simulink model "heldreset"  (R2022b)
settings: Solver=FixedStepDiscrete  StartTime=0.0  StopTime=10.0  FixedStep=0.1  RelTol=1e-3
settings Model: Creator=ahmed  LastModifiedBy=ahmed

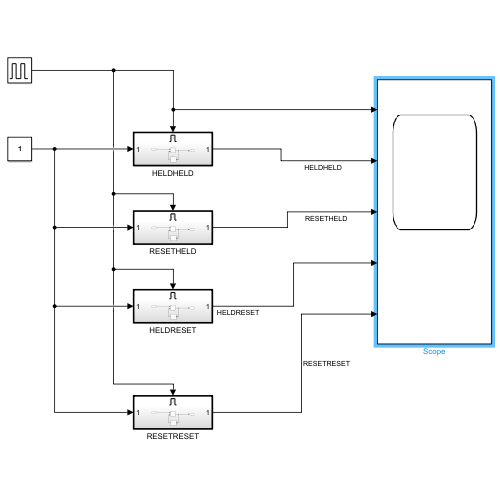
[thumbnail: Simulink's stored preview of the top-level diagram]
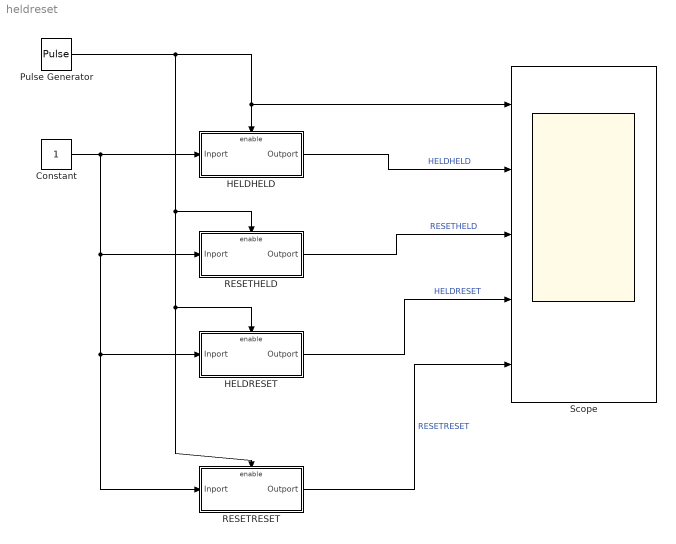
== system heldreset ==
  Constant : Constant
  HELDHELD : Subsystem  TreatAsAtomicUnit=on
  HELDRESET : Subsystem  TreatAsAtomicUnit=on
  Pulse Generator : DiscretePulseGenerator  PulseType=Time based  Period=1  PulseWidth=50
  RESETHELD : Subsystem  TreatAsAtomicUnit=on
  RESETRESET : Subsystem  TreatAsAtomicUnit=on
  Scope : Scope  NumInputPorts=5
  wires:
  Constant/1 -> HELDHELD/1(Inport), HELDRESET/1(Inport), RESETRESET/1(Inport), RESETHELD/1(Inport)
  Pulse Generator/1 -> RESETHELD/Enable, HELDRESET/Enable, RESETRESET/Enable, HELDHELD/Enable, Scope/1
  HELDHELD/1(Outport) -> Scope/2  "HELDHELD"
  RESETHELD/1(Outport) -> Scope/3  "RESETHELD"
  RESETRESET/1(Outport) -> Scope/5  "RESETRESET"
  HELDRESET/1(Outport) -> Scope/4  "HELDRESET"

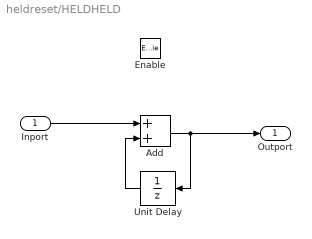
== system heldreset/HELDHELD ==
  Inport : Inport
  Enable : EnablePort
  Add : Sum
  Unit Delay : UnitDelay  SampleTime=-1  HasFrameUpgradeWarning=on
  Outport : Outport
  wires:
  Unit Delay/1 -> Add/2
  Add/1 -> Outport/1, Unit Delay/1
  Inport/1 -> Add/1

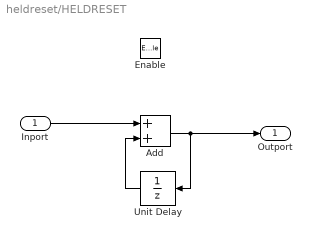
== system heldreset/HELDRESET ==
  Inport : Inport
  Enable : EnablePort
  Add : Sum
  Unit Delay : UnitDelay  SampleTime=-1  HasFrameUpgradeWarning=on
  Outport : Outport  OutputWhenDisabled=reset  InitialOutput=0
  wires:
  Inport/1 -> Add/1
  Add/1 -> Unit Delay/1, Outport/1
  Unit Delay/1 -> Add/2

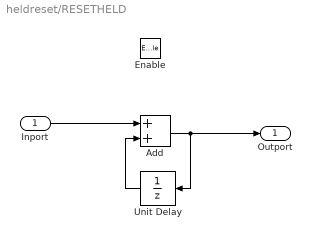
== system heldreset/RESETHELD ==
  Inport : Inport
  Enable : EnablePort  StatesWhenEnabling=reset
  Add : Sum
  Unit Delay : UnitDelay  SampleTime=-1  HasFrameUpgradeWarning=on
  Outport : Outport
  wires:
  Inport/1 -> Add/1
  Add/1 -> Unit Delay/1, Outport/1
  Unit Delay/1 -> Add/2

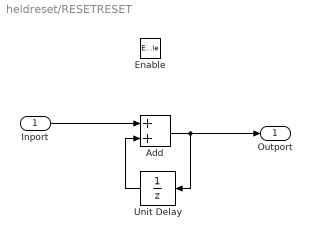
== system heldreset/RESETRESET ==
  Inport : Inport
  Enable : EnablePort  StatesWhenEnabling=reset
  Add : Sum
  Unit Delay : UnitDelay  SampleTime=-1  HasFrameUpgradeWarning=on
  Outport : Outport  OutputWhenDisabled=reset  InitialOutput=0
  wires:
  Unit Delay/1 -> Add/2
  Add/1 -> Outport/1, Unit Delay/1
  Inport/1 -> Add/1
